simulink model "multi_model_attitude_controller1_1"  (R2016b)
settings: Solver=ode15s  StartTime=0.0  StopTime=inf  FixedStep=0.001  MaxStep=0.004  RelTol=1e-3
InitFcn:
  | kR_old=0;
  | kOm_old=0;
undefined symbols (not defined in the file or in its folder): deg, rad, s
libraries: simulink x32, aerolibconvert2 x6, aerolibobsolete x2, aerolibtransform2 x2, aerolibatmos2 x2, aerolibnav x2, aerolibanimutils x2
(part 2 of 3)

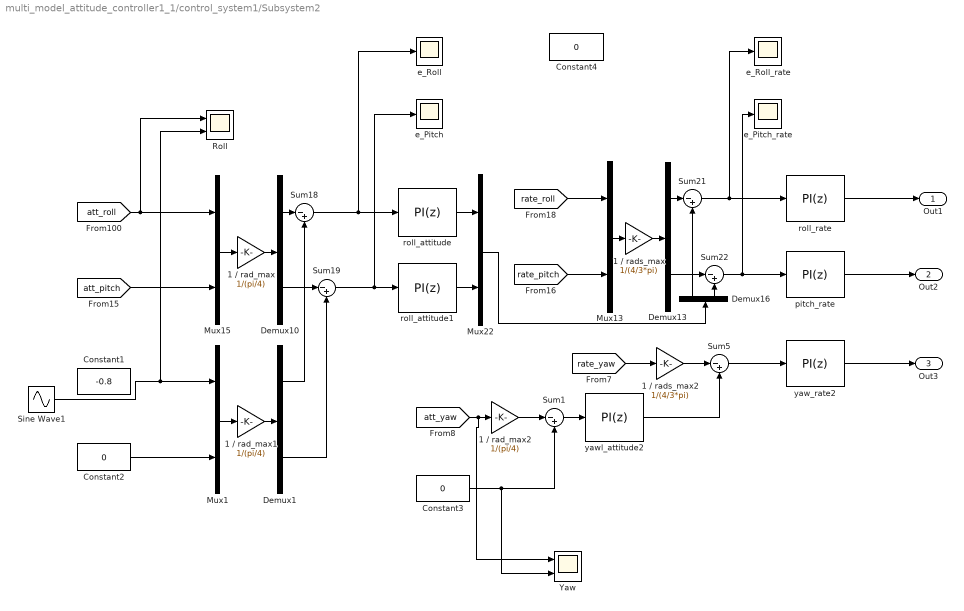
== system multi_model_attitude_controller1_1/control_system1/Subsystem2 ==
  1 / rad_max : Gain  Gain=1/(pi/4)
  1 / rad_max1 : Gain  Gain=1/(pi/4)
  1 / rad_max2 : Gain  Gain=1/(pi/4)
  1 / rads_max : Gain  Gain=1/(4/3*pi)
  1 / rads_max2 : Gain  Gain=1/(4/3*pi)
  Constant1 : Constant  Value=-0.8  SampleTime=0.004
  Constant2 : Constant  Value=0  SampleTime=0.004
  Constant3 : Constant  Value=0  SampleTime=0.004
  Constant4 : Constant  Value=0  SampleTime=0.004
  Demux{1,10,13,16} (4 alike) : Demux  Outputs=2
  Mux{1,13,15,22} (4 alike) : Mux  Inputs=2
  Roll : Scope  NumInputPorts=2
  Sine Wave1 : Sin  Amplitude=pi/9  Frequency=pi  Phase=pi/2  SampleTime=0.004
  Sum{1,5,18..19,21..22} (6 alike) : Sum  Inputs=|-+
  Yaw : Scope  NumInputPorts=2
  e_Pitch : Scope
  e_Pitch_rate : Scope
  e_Roll : Scope
  e_Roll_rate : Scope
  pitch_rate : simulink/Continuous/PID Controller  Controller=PI  TimeDomain=Discrete-time  SampleTime=-1  IntegratorMethod=Forward Euler  FilterMethod=Forward Euler  Form=Parallel  UseFilter=on  ControllerParametersSource=internal  P=0.266243984189179  I=1.55321106287276  D=0.0024  N=100  InitialConditionSource=internal  InitialConditionForIntegrator=0  InitialConditionForFilter=0  ExternalReset=none  LimitOutput=on  UpperSaturationLimit=1  LowerSaturationLimit=-1  LinearizeAsGain=on  AntiWindupMode=none  Kb=1  TrackingMode=off  Kt=1  PParamMin=[]  PParamMax=[]  IParamMin=[]  IParamMax=[]  DParamMin=[]  DParamMax=[]  NParamMin=[]  NParamMax=[]  KbParamMin=[]  KbParamMax=[]  KtParamMin=[]  KtParamMax=[]  POutMin=[]  POutMax=[]  IOutMin=[]  IOutMax=[]  DOutMin=[]  DOutMax=[]  NOutMin=[]  NOutMax=[]  KbOutMin=[]  KbOutMax=[]  KtOutMin=[]  KtOutMax=[]  IntegratorOutMin=[]  IntegratorOutMax=[]  FilterOutMin=[]  FilterOutMax=[]  SumOutMin=[]  SumOutMax=[]  SumI1OutMin=[]  SumI1OutMax=[]  SumI2OutMin=[]  SumI2OutMax=[]  SumI3OutMin=[]  SumI3OutMax=[]  SumDOutMin=[]  SumDOutMax=[]  SaturationOutMin=[]  SaturationOutMax=[]  IntegratorContinuousStateAttributes=''  IntegratorStateMustResolveToSignalObject=off  IntegratorRTWStateStorageClass=Auto  FilterContinuousStateAttributes=''  FilterStateMustResolveToSignalObject=off  FilterRTWStateStorageClass=Auto  DifferentiatorICPrevScaledInput=0  DifferentiatorOutMin=[]  DifferentiatorOutMax=[]
  roll_attitude : simulink/Continuous/PID Controller  Controller=PI  TimeDomain=Discrete-time  SampleTime=-1  IntegratorMethod=Forward Euler  FilterMethod=Forward Euler  Form=Parallel  UseFilter=on  ControllerParametersSource=internal  P=1.14248027715292  I=2.67479021353904  D=0.01  N=100  InitialConditionSource=internal  InitialConditionForIntegrator=0  InitialConditionForFilter=0  ExternalReset=none  LimitOutput=on  UpperSaturationLimit=1  LowerSaturationLimit=-1  LinearizeAsGain=on  AntiWindupMode=none  Kb=1  TrackingMode=off  Kt=1  PParamMin=[]  PParamMax=[]  IParamMin=[]  IParamMax=[]  DParamMin=[]  DParamMax=[]  NParamMin=[]  NParamMax=[]  KbParamMin=[]  KbParamMax=[]  KtParamMin=[]  KtParamMax=[]  POutMin=[]  POutMax=[]  IOutMin=[]  IOutMax=[]  DOutMin=[]  DOutMax=[]  NOutMin=[]  NOutMax=[]  KbOutMin=[]  KbOutMax=[]  KtOutMin=[]  KtOutMax=[]  IntegratorOutMin=[]  IntegratorOutMax=[]  FilterOutMin=[]  FilterOutMax=[]  SumOutMin=[]  SumOutMax=[]  SumI1OutMin=[]  SumI1OutMax=[]  SumI2OutMin=[]  SumI2OutMax=[]  SumI3OutMin=[]  SumI3OutMax=[]  SumDOutMin=[]  SumDOutMax=[]  SaturationOutMin=[]  SaturationOutMax=[]  IntegratorContinuousStateAttributes=''  IntegratorStateMustResolveToSignalObject=off  IntegratorRTWStateStorageClass=Auto  FilterContinuousStateAttributes=''  FilterStateMustResolveToSignalObject=off  FilterRTWStateStorageClass=Auto  DifferentiatorICPrevScaledInput=0  DifferentiatorOutMin=[]  DifferentiatorOutMax=[]
  roll_attitude1 : simulink/Continuous/PID Controller  Controller=PI  TimeDomain=Discrete-time  SampleTime=-1  IntegratorMethod=Forward Euler  FilterMethod=Forward Euler  Form=Parallel  UseFilter=on  ControllerParametersSource=internal  P=1.14248027709528  I=2.67479021340165  D=0.01  N=100  InitialConditionSource=internal  InitialConditionForIntegrator=0  InitialConditionForFilter=0  ExternalReset=none  LimitOutput=on  UpperSaturationLimit=1  LowerSaturationLimit=-1  LinearizeAsGain=on  AntiWindupMode=none  Kb=1  TrackingMode=off  Kt=1  PParamMin=[]  PParamMax=[]  IParamMin=[]  IParamMax=[]  DParamMin=[]  DParamMax=[]  NParamMin=[]  NParamMax=[]  KbParamMin=[]  KbParamMax=[]  KtParamMin=[]  KtParamMax=[]  POutMin=[]  POutMax=[]  IOutMin=[]  IOutMax=[]  DOutMin=[]  DOutMax=[]  NOutMin=[]  NOutMax=[]  KbOutMin=[]  KbOutMax=[]  KtOutMin=[]  KtOutMax=[]  IntegratorOutMin=[]  IntegratorOutMax=[]  FilterOutMin=[]  FilterOutMax=[]  SumOutMin=[]  SumOutMax=[]  SumI1OutMin=[]  SumI1OutMax=[]  SumI2OutMin=[]  SumI2OutMax=[]  SumI3OutMin=[]  SumI3OutMax=[]  SumDOutMin=[]  SumDOutMax=[]  SaturationOutMin=[]  SaturationOutMax=[]  IntegratorContinuousStateAttributes=''  IntegratorStateMustResolveToSignalObject=off  IntegratorRTWStateStorageClass=Auto  FilterContinuousStateAttributes=''  FilterStateMustResolveToSignalObject=off  FilterRTWStateStorageClass=Auto  DifferentiatorICPrevScaledInput=0  DifferentiatorOutMin=[]  DifferentiatorOutMax=[]
  roll_rate : simulink/Continuous/PID Controller  Controller=PI  TimeDomain=Discrete-time  SampleTime=-1  IntegratorMethod=Forward Euler  FilterMethod=Forward Euler  Form=Parallel  UseFilter=on  ControllerParametersSource=internal  P=0.327684903617463  I=1.91164438507472  D=0.0024  N=100  InitialConditionSource=internal  InitialConditionForIntegrator=0  InitialConditionForFilter=0  ExternalReset=none  LimitOutput=on  UpperSaturationLimit=1  LowerSaturationLimit=-1  LinearizeAsGain=on  AntiWindupMode=none  Kb=1  TrackingMode=off  Kt=1  PParamMin=[]  PParamMax=[]  IParamMin=[]  IParamMax=[]  DParamMin=[]  DParamMax=[]  NParamMin=[]  NParamMax=[]  KbParamMin=[]  KbParamMax=[]  KtParamMin=[]  KtParamMax=[]  POutMin=[]  POutMax=[]  IOutMin=[]  IOutMax=[]  DOutMin=[]  DOutMax=[]  NOutMin=[]  NOutMax=[]  KbOutMin=[]  KbOutMax=[]  KtOutMin=[]  KtOutMax=[]  IntegratorOutMin=[]  IntegratorOutMax=[]  FilterOutMin=[]  FilterOutMax=[]  SumOutMin=[]  SumOutMax=[]  SumI1OutMin=[]  SumI1OutMax=[]  SumI2OutMin=[]  SumI2OutMax=[]  SumI3OutMin=[]  SumI3OutMax=[]  SumDOutMin=[]  SumDOutMax=[]  SaturationOutMin=[]  SaturationOutMax=[]  IntegratorContinuousStateAttributes=''  IntegratorStateMustResolveToSignalObject=off  IntegratorRTWStateStorageClass=Auto  FilterContinuousStateAttributes=''  FilterStateMustResolveToSignalObject=off  FilterRTWStateStorageClass=Auto  DifferentiatorICPrevScaledInput=0  DifferentiatorOutMin=[]  DifferentiatorOutMax=[]
  yaw_rate2 : simulink/Continuous/PID Controller  Controller=PI  TimeDomain=Discrete-time  SampleTime=-1  IntegratorMethod=Forward Euler  FilterMethod=Forward Euler  Form=Parallel  UseFilter=on  ControllerParametersSource=internal  P=0.3  I=0.03  D=0.0024  N=100  InitialConditionSource=internal  InitialConditionForIntegrator=0  InitialConditionForFilter=0  ExternalReset=none  LimitOutput=on  UpperSaturationLimit=1  LowerSaturationLimit=-1  LinearizeAsGain=on  AntiWindupMode=none  Kb=1  TrackingMode=off  Kt=1  PParamMin=[]  PParamMax=[]  IParamMin=[]  IParamMax=[]  DParamMin=[]  DParamMax=[]  NParamMin=[]  NParamMax=[]  KbParamMin=[]  KbParamMax=[]  KtParamMin=[]  KtParamMax=[]  POutMin=[]  POutMax=[]  IOutMin=[]  IOutMax=[]  DOutMin=[]  DOutMax=[]  NOutMin=[]  NOutMax=[]  KbOutMin=[]  KbOutMax=[]  KtOutMin=[]  KtOutMax=[]  IntegratorOutMin=[]  IntegratorOutMax=[]  FilterOutMin=[]  FilterOutMax=[]  SumOutMin=[]  SumOutMax=[]  SumI1OutMin=[]  SumI1OutMax=[]  SumI2OutMin=[]  SumI2OutMax=[]  SumI3OutMin=[]  SumI3OutMax=[]  SumDOutMin=[]  SumDOutMax=[]  SaturationOutMin=[]  SaturationOutMax=[]  IntegratorContinuousStateAttributes=''  IntegratorStateMustResolveToSignalObject=off  IntegratorRTWStateStorageClass=Auto  FilterContinuousStateAttributes=''  FilterStateMustResolveToSignalObject=off  FilterRTWStateStorageClass=Auto  DifferentiatorICPrevScaledInput=0  DifferentiatorOutMin=[]  DifferentiatorOutMax=[]
  yawl_attitude2 : simulink/Continuous/PID Controller  Controller=PI  TimeDomain=Discrete-time  SampleTime=-1  IntegratorMethod=Forward Euler  FilterMethod=Forward Euler  Form=Parallel  UseFilter=on  ControllerParametersSource=internal  P=0.5  I=0.05  D=0.01  N=100  InitialConditionSource=internal  InitialConditionForIntegrator=0  InitialConditionForFilter=0  ExternalReset=none  LimitOutput=on  UpperSaturationLimit=1  LowerSaturationLimit=-1  LinearizeAsGain=on  AntiWindupMode=none  Kb=1  TrackingMode=off  Kt=1  PParamMin=[]  PParamMax=[]  IParamMin=[]  IParamMax=[]  DParamMin=[]  DParamMax=[]  NParamMin=[]  NParamMax=[]  KbParamMin=[]  KbParamMax=[]  KtParamMin=[]  KtParamMax=[]  POutMin=[]  POutMax=[]  IOutMin=[]  IOutMax=[]  DOutMin=[]  DOutMax=[]  NOutMin=[]  NOutMax=[]  KbOutMin=[]  KbOutMax=[]  KtOutMin=[]  KtOutMax=[]  IntegratorOutMin=[]  IntegratorOutMax=[]  FilterOutMin=[]  FilterOutMax=[]  SumOutMin=[]  SumOutMax=[]  SumI1OutMin=[]  SumI1OutMax=[]  SumI2OutMin=[]  SumI2OutMax=[]  SumI3OutMin=[]  SumI3OutMax=[]  SumDOutMin=[]  SumDOutMax=[]  SaturationOutMin=[]  SaturationOutMax=[]  IntegratorContinuousStateAttributes=''  IntegratorStateMustResolveToSignalObject=off  IntegratorRTWStateStorageClass=Auto  FilterContinuousStateAttributes=''  FilterStateMustResolveToSignalObject=off  FilterRTWStateStorageClass=Auto  DifferentiatorICPrevScaledInput=0  DifferentiatorOutMin=[]  DifferentiatorOutMax=[]
  Out1 : Outport
  Out2 : Outport  Port=2
  Out3 : Outport  Port=3
  wires:
  Sine Wave1/1 -> Roll/2, Mux1/1
  Mux1/1 -> 1 / rad_max1/1
  Constant2/1 -> Mux1/2
  Demux1/1 -> Sum18/2
  Mux22/1 -> Demux16/1
  yaw_rate2/1 -> Out3/1
  Sum5/1 -> yaw_rate2/1
  yawl_attitude2/1 -> Sum5/2
  1 / rad_max2/1 -> Sum1/1
  [att_yaw] -> Yaw/1, 1 / rad_max2/1
  1 / rads_max2/1 -> Sum5/1
  [rate_yaw] -> 1 / rads_max2/1
  1 / rad_max/1 -> Demux10/1
  Demux10/1 -> Sum18/1
  Demux16/2 -> Sum22/2
  roll_attitude1/1 -> Mux22/2
  Demux13/2 -> Sum22/1
  Sum21/1 -> e_Roll_rate/1, roll_rate/1
  Sum22/1 -> e_Pitch_rate/1, pitch_rate/1
  roll_attitude/1 -> Mux22/1
  [rate_pitch] -> Mux13/2
  Demux10/2 -> Sum19/1
  [att_pitch] -> Mux15/2
  [rate_roll] -> Mux13/1
  1 / rads_max/1 -> Demux13/1
  Sum18/1 -> e_Roll/1, roll_attitude/1
  Mux13/1 -> 1 / rads_max/1
  Demux13/1 -> Sum21/1
  Sum19/1 -> e_Pitch/1, roll_attitude1/1
  Mux15/1 -> 1 / rad_max/1
  [att_roll] -> Roll/1, Mux15/1
  roll_rate/1 -> Out1/1
  pitch_rate/1 -> Out2/1
  1 / rad_max1/1 -> Demux1/1
  Demux1/2 -> Sum19/2
  Sum1/1 -> yawl_attitude2/1
  Constant3/1 -> Yaw/2, Sum1/2
  Demux16/1 -> Sum21/2

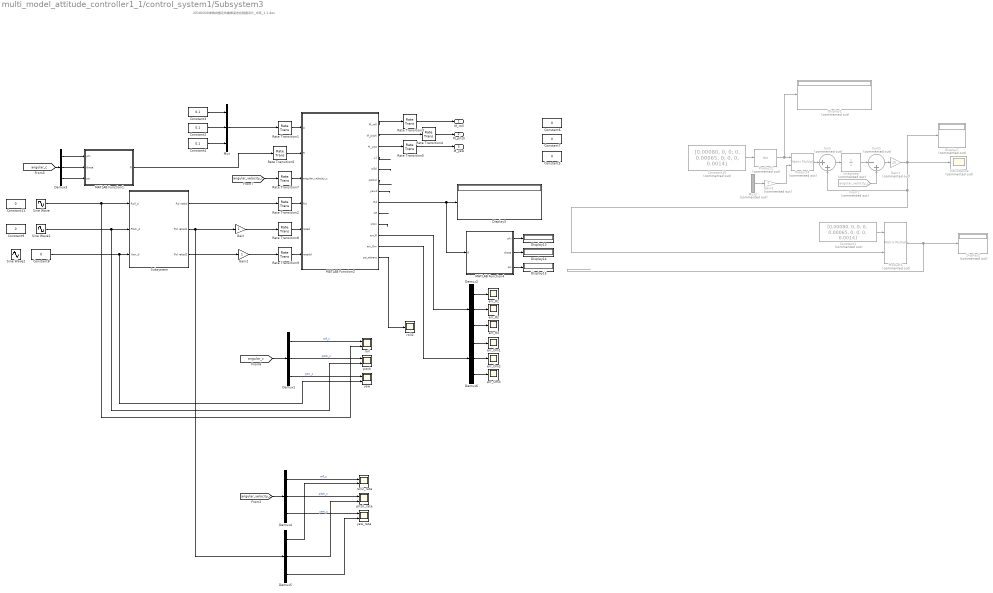
== system multi_model_attitude_controller1_1/control_system1/Subsystem3 ==
  note: 20180328 参数自整定的鲁棒姿态控制器设计_中英_1.1.doc
  Constant1 : Constant  Commented=on  Value=[0.00080, 0, 0; 0, 0.00065, 0; 0, 0, 0.0014]  SampleTime=0.004
  Constant10 : Constant  Commented=on  Value=[0.00080, 0, 0; 0, 0.00065, 0; 0, 0, 0.0014]  SampleTime=0.004
  Constant{5..9,11} (6 alike) : Constant  Value=0  SampleTime=0.004
  Constant2 : Constant  Value=0.1  SampleTime=0.004
  Constant3 : Constant  Value=0.1  SampleTime=0.004
  Constant4 : Constant  Value=0.1  SampleTime=0.004
  Demux{1..6} (6 alike) : Demux  Outputs=3
  Display1 : Display  Commented=on
  Display{3,13..15} (4 alike) : Display
  Display2 : Display  Commented=on
  Display7 : Display  Commented=on
  From1 : From  Commented=on  GotoTag=angular_velocity_c  TagVisibility=global
  Gain : Gain
  Gain1 : Gain  Commented=on  Gain=20
  Gain2 : Gain
  Gain3 : Gain  Commented=on
  Integrator : Integrator  Commented=on
  MATLAB Function1 : MATLAB Function  TreatAsAtomicUnit=on
  MATLAB Function2 : MATLAB Function  TreatAsAtomicUnit=on
  MATLAB Function4 : MATLAB Function  TreatAsAtomicUnit=on
  Mux : Mux  Inputs=3
  Mux2 : Mux  Commented=on  Inputs=3
  Product1 : Product  Commented=on  Multiplication=Matrix(*)
  Product2 : Product  Commented=on  Inputs=/  Multiplication=Matrix(*)
  Product4 : Product  Commented=on  Multiplication=Matrix(*)
  Rate Transition{1..9} (9 alike) : RateTransition  OutPortSampleTime=0.004
  Sine Wave : Sin  Amplitude=pi/9  Frequency=pi  SampleTime=0.004
  Sine Wave1 : Sin  Amplitude=pi/9  Frequency=pi  Phase=pi/2  SampleTime=0.004
  Sine Wave2 : Sin  Amplitude=pi/9  Frequency=pi  SampleTime=0.004
  Subsystem : Subsystem
  Sum : Sum  Commented=on  Inputs=|++
  Sum1 : Sum  Commented=on  Inputs=|-+
  disturbance : Scope  Commented=on
  err_Om1 : Scope
  err_Om2 : Scope
  err_Om3 : Scope
  err_R1 : Scope
  err_R2 : Scope
  err_R3 : Scope
  pitch : Scope  NumInputPorts=2
  pitch_rate : Scope  NumInputPorts=2
  roll : Scope  NumInputPorts=2
  roll2 : Scope
  roll2_rate : Scope  NumInputPorts=2
  yaw : Scope  NumInputPorts=2
  yaw_rate : Scope  NumInputPorts=2
  M_roll : Outport
  M_pitch : Outport  Port=2
  M_yaw : Outport  Port=3
  wires:
  Gain3/1 -> Product4/2
  Product1/1 -> Display2/1
  Rate Transition5/1 -> M_yaw/1
  Rate Transition4/1 -> M_pitch/1
  Rate Transition3/1 -> M_roll/1
  Constant1/1 -> Product1/1
  Rate Transition2/1 -> MATLAB Function2/4("Rd ")
  Constant2/1 -> Mux/2
  From1/1 -> Sum1/2
  Gain1/1 -> Display7/1, disturbance/1, Sum/2, Product1/2
  Mux/1 -> Rate Transition1/1
  Constant10/1 -> Product2/1
  Product2/1 -> Product4/1, Display1/1
  MATLAB Function2/3(M_yaw) -> Rate Transition5/1
  Sine Wave/1 -> roll/2, Subsystem/1(Roll_d)
  Sum1/1 -> Gain1/1
  MATLAB Function2/1(M_roll) -> Rate Transition3/1
  Sum/1 -> Integrator/1
  Product4/1 -> Sum/1
  Constant3/1 -> Mux/1
  MATLAB Function2/2(M_pitch) -> Rate Transition4/1
  Subsystem/1(Rd rated) -> Rate Transition2/1
  Constant4/1 -> Mux/3
  Mux2/1 -> Gain3/1
  Integrator/1 -> Sum1/1
  Rate Transition6/1 -> MATLAB Function2/2(R)
  Demux1/3 -> yaw/1  "yaw_c"
  Rate Transition7/1 -> MATLAB Function2/3(angular_velocity_c)
  Demux1/1 -> roll/1  "roll_c"
  Rate Transition1/1 -> MATLAB Function2/1(A)
  [angular_velocity_c] -> Rate Transition7/1
  MATLAB Function1/1(R) -> Rate Transition6/1
  Demux1/2 -> pitch/1  "pitch_c"
  MATLAB Function2/5(rolld) -> ?
  MATLAB Function2/7(yawd) -> ?
  MATLAB Function2/6(pitchd) -> ?
  MATLAB Function2/4(u1) -> ?
  Demux2/1 -> err_R1/1
  MATLAB Function2/9(kR) -> ?
  MATLAB Function2/10(kOm) -> ?
  Demux2/2 -> err_R2/1
  Demux2/3 -> err_R3/1
  Constant8/1 -> yaw/2, Subsystem/3(Yaw_d)
  Sine Wave1/1 -> pitch/2, Subsystem/2(PItch_d)
  MATLAB Function4/1(phi) -> Display13/1
  MATLAB Function4/2(theta) -> Display14/1
  MATLAB Function4/3(psi) -> Display15/1
  MATLAB Function2/8(Rd) -> MATLAB Function4/1(R), Display3/1
  [angular_c] -> Demux1/1
  Demux3/2 -> MATLAB Function1/2(theta)
  Demux3/1 -> MATLAB Function1/1(phi)
  Demux3/3 -> MATLAB Function1/3(psi)
  Rate Transition8/1 -> MATLAB Function2/5(rated)
  Rate Transition9/1 -> MATLAB Function2/6(ratedd)
  Subsystem/2(Rd rated1) -> Demux5/1, Gain/1
  Subsystem/3(Rd rated2) -> Gain2/1
  Demux4/3 -> yaw_rate/1  "yaw_c"
  Demux4/1 -> roll2_rate/1  "roll_c"
  Demux4/2 -> pitch_rate/1  "pitch_c"
  [angular_velocity_c] -> Demux4/1
  Demux5/1 -> roll2_rate/2
  Demux5/2 -> pitch_rate/2
  Demux5/3 -> yaw_rate/2
  [angular_c] -> Demux3/1
  MATLAB Function2/13(psi_attract) -> roll2/1
  MATLAB Function2/11(err_R) -> Demux2/1
  Demux6/1 -> err_Om1/1
  Demux6/2 -> err_Om2/1
  Demux6/3 -> err_Om3/1
  MATLAB Function2/12(err_Om) -> Demux6/1
  Gain/1 -> Rate Transition8/1
  Gain2/1 -> Rate Transition9/1

== system multi_model_attitude_controller1_1/dynamic_model1/normalize ==
  pwm1 : Inport
  pwm2 : Inport  Port=2
  pwm3 : Inport  Port=3
  pwm4 : Inport  Port=4
  pwm5 : Inport  Port=5
  pwm6 : Inport  Port=6
  pwm7 : Inport  Port=7
  pwm8 : Inport  Port=8
  Mux5 : Mux  Inputs=8
  Saturation{,3..9} (8 alike) : Saturate  UpperLimit=1  LowerLimit=0
  voltage{1..8} (8 alike) : Fcn  Expr=(u-1000)/1000
  normalized_signals : Outport
  wires:
  Saturation5/1 -> Mux5/4
  Saturation7/1 -> Mux5/6
  voltage6/1 -> Saturation7/1
  voltage5/1 -> Saturation5/1
  voltage2/1 -> Saturation/1
  voltage7/1 -> Saturation8/1
  Saturation8/1 -> Mux5/7
  voltage8/1 -> Saturation9/1
  Saturation9/1 -> Mux5/8
  pwm3/1 -> voltage4/1
  Mux5/1 -> normalized_signals/1
  pwm1/1 -> voltage2/1
  voltage4/1 -> Saturation4/1
  Saturation4/1 -> Mux5/3
  pwm7/1 -> voltage7/1
  pwm6/1 -> voltage6/1
  pwm8/1 -> voltage8/1
  pwm4/1 -> voltage5/1
  pwm5/1 -> voltage1/1
  pwm2/1 -> voltage3/1
  voltage1/1 -> Saturation6/1
  Saturation6/1 -> Mux5/5
  Saturation/1 -> Mux5/1
  Saturation3/1 -> Mux5/2
  voltage3/1 -> Saturation3/1

== system multi_model_attitude_controller1_1/dynamic_model1/transfer_function ==
  load : Inport  PortDimensions=[8]
  voltage : Inport  Port=2  PortDimensions=[8]
  Demux13 : Demux  Outputs=8
  Mux4 : Mux  Inputs=8
  Product : Product
  Transfer Fcn{1..8} (8 alike) : TransferFcn  Numerator=[325]  Denominator=[2.5e-08 0.01 1]  ContinuousStateAttributes='angular_velocity'
  thrust : Outport
  wires:
  Demux13/6 -> Transfer Fcn6/1
  Transfer Fcn4/1 -> Mux4/4
  Transfer Fcn2/1 -> Mux4/3
  Demux13/8 -> Transfer Fcn8/1
  Transfer Fcn8/1 -> Mux4/8
  Transfer Fcn1/1 -> Mux4/2
  Demux13/7 -> Transfer Fcn7/1
  Transfer Fcn7/1 -> Mux4/7
  Transfer Fcn5/1 -> Mux4/5
  Demux13/5 -> Transfer Fcn5/1
  Transfer Fcn3/1 -> Mux4/1
  Transfer Fcn6/1 -> Mux4/6
  Demux13/1 -> Transfer Fcn3/1
  Demux13/2 -> Transfer Fcn1/1
  Demux13/3 -> Transfer Fcn2/1
  Demux13/4 -> Transfer Fcn4/1
  voltage/1 -> Product/2
  Product/1 -> Demux13/1
  Mux4/1 -> thrust/1
  load/1 -> Product/1

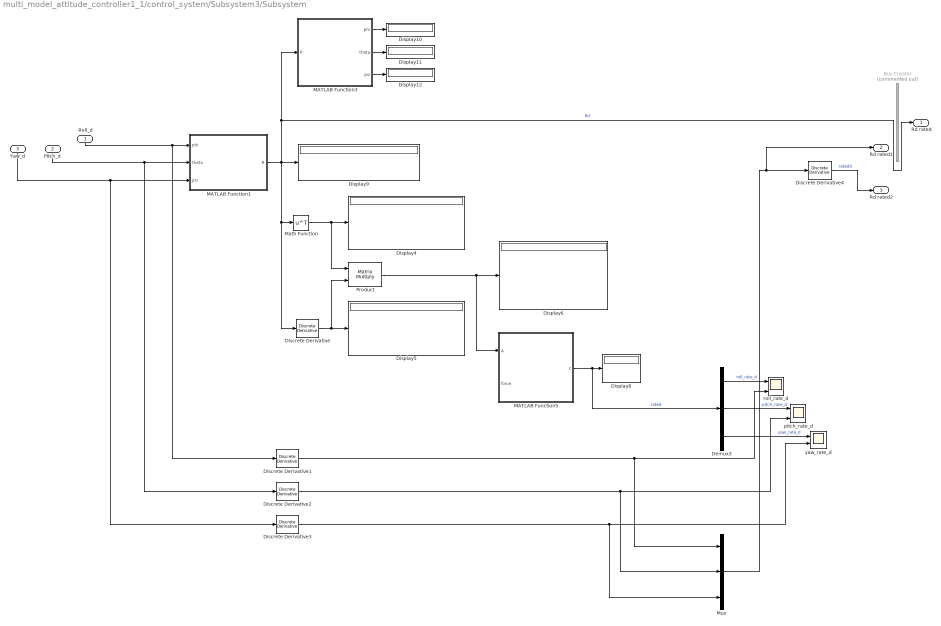
== system multi_model_attitude_controller1_1/control_system/Subsystem3/Subsystem ==
  Roll_d : Inport
  PItch_d : Inport  Port=2
  Yaw_d : Inport  Port=3
  Bus Creator : BusCreator  Commented=on  Inputs=3
  Demux3 : Demux  Outputs=3
  Discrete Derivative{,1..4} (5 alike) : simulink/Discrete/Discrete Derivative  gainval=1.0  ICPrevScaledInput=0.0  OutMin=[]  OutMax=[]  OutDataType=fixdt(1, 16)  OutScaling=2^-10  DoSatur=off
  Display{4..6,8..12} (8 alike) : Display
  MATLAB Function1 : MATLAB Function  TreatAsAtomicUnit=on
  MATLAB Function3 : MATLAB Function  TreatAsAtomicUnit=on
  MATLAB Function5 : MATLAB Function  TreatAsAtomicUnit=on
  Math Function : Math  Operator=transpose  SaturateOnIntegerOverflow=on
  Mux : Mux  Inputs=3
  Product : Product  Multiplication=Matrix(*)
  pitch_rate_d : Scope  NumInputPorts=2
  roll_rate_d : Scope  NumInputPorts=2
  yaw_rate_d : Scope  NumInputPorts=2
  Rd rated : Outport
  Rd rated1 : Outport  Port=2
  Rd rated2 : Outport  Port=3
  wires:
  Discrete Derivative3/1 -> yaw_rate_d/2, Mux/3
  MATLAB Function3/2(theta) -> Display11/1
  Discrete Derivative1/1 -> roll_rate_d/2, Mux/1
  Discrete Derivative2/1 -> pitch_rate_d/2, Mux/2
  Product/1 -> MATLAB Function5/1(A), Display6/1
  Discrete Derivative/1 -> Product/2, Display5/1
  MATLAB Function1/1(R) -> Rd rated/1, MATLAB Function3/1(R), Display9/1, Math Function/1, Discrete Derivative/1  "Rd"
  MATLAB Function3/1(phi) -> Display10/1
  MATLAB Function3/3(psi) -> Display12/1
  Math Function/1 -> Product/1, Display4/1
  MATLAB Function5/1(t) -> Demux3/1, Display8/1  "rated"
  Demux3/3 -> yaw_rate_d/1  "yaw_rate_d"
  Demux3/1 -> roll_rate_d/1  "roll_rate_d"
  Demux3/2 -> pitch_rate_d/1  "pitch_rate_d"
  Roll_d/1 -> Discrete Derivative1/1, MATLAB Function1/1(phi)
  ? -> MATLAB Function5/2(force)
  Yaw_d/1 -> Discrete Derivative3/1, MATLAB Function1/3(psi)
  PItch_d/1 -> Discrete Derivative2/1, MATLAB Function1/2(theta)
  Discrete Derivative4/1 -> Rd rated2/1  "ratedd"
  Mux/1 -> Rd rated1/1, Discrete Derivative4/1

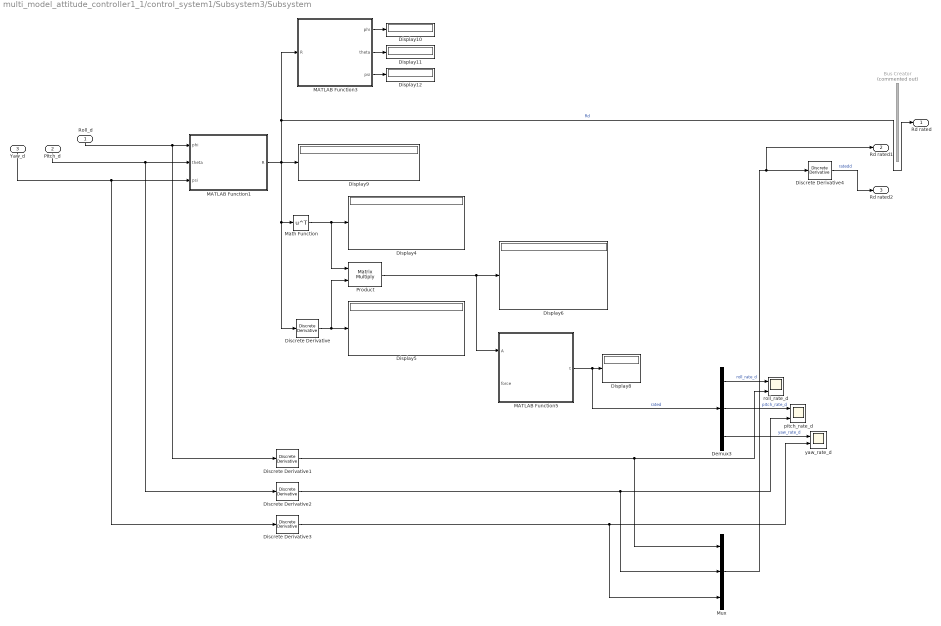
== system multi_model_attitude_controller1_1/control_system1/Subsystem3/Subsystem ==
  Roll_d : Inport
  PItch_d : Inport  Port=2
  Yaw_d : Inport  Port=3
  Bus Creator : BusCreator  Commented=on  Inputs=3
  Demux3 : Demux  Outputs=3
  Discrete Derivative{,1..4} (5 alike) : simulink/Discrete/Discrete Derivative  gainval=1.0  ICPrevScaledInput=0.0  OutMin=[]  OutMax=[]  OutDataType=fixdt(1, 16)  OutScaling=2^-10  DoSatur=off
  Display{4..6,8..12} (8 alike) : Display
  MATLAB Function1 : MATLAB Function  TreatAsAtomicUnit=on
  MATLAB Function3 : MATLAB Function  TreatAsAtomicUnit=on
  MATLAB Function5 : MATLAB Function  TreatAsAtomicUnit=on
  Math Function : Math  Operator=transpose  SaturateOnIntegerOverflow=on
  Mux : Mux  Inputs=3
  Product : Product  Multiplication=Matrix(*)
  pitch_rate_d : Scope  NumInputPorts=2
  roll_rate_d : Scope  NumInputPorts=2
  yaw_rate_d : Scope  NumInputPorts=2
  Rd rated : Outport
  Rd rated1 : Outport  Port=2
  Rd rated2 : Outport  Port=3
  wires:
  Discrete Derivative3/1 -> yaw_rate_d/2, Mux/3
  MATLAB Function3/2(theta) -> Display11/1
  Discrete Derivative1/1 -> roll_rate_d/2, Mux/1
  Discrete Derivative2/1 -> pitch_rate_d/2, Mux/2
  Product/1 -> MATLAB Function5/1(A), Display6/1
  Discrete Derivative/1 -> Product/2, Display5/1
  MATLAB Function1/1(R) -> Rd rated/1, MATLAB Function3/1(R), Display9/1, Math Function/1, Discrete Derivative/1  "Rd"
  MATLAB Function3/1(phi) -> Display10/1
  MATLAB Function3/3(psi) -> Display12/1
  Math Function/1 -> Product/1, Display4/1
  MATLAB Function5/1(t) -> Demux3/1, Display8/1  "rated"
  Demux3/3 -> yaw_rate_d/1  "yaw_rate_d"
  Demux3/1 -> roll_rate_d/1  "roll_rate_d"
  Demux3/2 -> pitch_rate_d/1  "pitch_rate_d"
  Roll_d/1 -> Discrete Derivative1/1, MATLAB Function1/1(phi)
  ? -> MATLAB Function5/2(force)
  Yaw_d/1 -> Discrete Derivative3/1, MATLAB Function1/3(psi)
  PItch_d/1 -> Discrete Derivative2/1, MATLAB Function1/2(theta)
  Discrete Derivative4/1 -> Rd rated2/1  "ratedd"
  Mux/1 -> Rd rated1/1, Discrete Derivative4/1

== matlab function multi_model_attitude_controller1_1/dynamic_model/MATLAB Function ==
  data: roll input; pitch input; altitude input; sonar_alt output
function sonar_alt = ultrasonic(roll, pitch, altitude)
if altitude > 0
    sonar_alt = sqrt(altitude^2 + (sqrt((altitude*tan(roll))^2 + (altitude*tan(pitch))^2))^2);
else
    sonar_alt = 0;
end

== matlab function multi_model_attitude_controller1_1/control_system1/Subsystem/MATLAB Function3 ==
  data: angular input; R output
function R = RPY_2_ZXY(angular)
%written by Daniel Mellinger
phi=angular(1);theta=angular(2);psi=angular(3);
% BRW = [ cos(psi)*cos(theta) - sin(phi)*sin(psi)*sin(theta), 
%     cos(theta)*sin(psi) + cos(psi)*sin(phi)*sin(theta), -cos(phi)*sin(theta)]
% 
% [                                 -cos(phi)*sin(psi),
%     cos(phi)*cos(psi),             sin(phi)]
% 
% [ cos(psi)*sin(theta) + cos(theta)*sin(phi)*sin(psi), 
%     sin(psi)*sin(theta) - cos(psi)*cos(theta)*sin(phi),
%     cos(phi)*cos(theta)]

R = [ cos(psi)*cos(theta) - sin(phi)*sin(psi)*sin(theta),... 
    cos(theta)*sin(psi) + cos(psi)*sin(phi)*sin(theta), -cos(phi)*sin(theta);...
    -cos(phi)*sin(psi),...
    cos(phi)*cos(psi),             sin(phi);...
    cos(psi)*sin(theta) + cos(theta)*sin(phi)*sin(psi),...
    sin(psi)*sin(theta) - cos(psi)*cos(theta)*sin(phi),...
    cos(phi)*cos(theta)];
    
    R = R';

== matlab function multi_model_attitude_controller1_1/control_system/Subsystem3/MATLAB Function2 ==
  data: A input; M_roll output; R input; angular_velocity_c input; M_pitch output; M_yaw output; u1 output; rolld output; pitchd output; yawd output; Rd output; kR output; kOm output; Rd input; err_R output; err_Om output; rated input; ratedd input; psi_attract output
function [M_roll, M_pitch,M_yaw,u1,rolld,pitchd,yawd,Rd,kR,kOm,err_R,err_Om,psi_attract] = attitude(A,R,angular_velocity_c,Rd,rated,ratedd)

 J = diag([0.00080, 0.00065, 0.0014]);
 J_ni=inv(J);
 e1 = [1;0;0];e2 = [0;1;0];e3 = [0;0;1];

Omega=angular_velocity_c;

Omegad = rated;
dOmegad = ratedd;

 b3c = A/norm(A);
 b3 = R(:,3);
 f = vec_dot(A,b3);
 u1=f;
    
%%%%%  姿态控制
 b1d = e1;
 b1c = -vec_cross(b3c,vec_cross(b3c,b1d));
 b1c = b1c/norm(vec_cross(b3c,b1d));
 Rc = [b1c vec_cross(b3c,b1c) b3c];
 

[rolld,pitchd,yawd]=RotToRPY_ZXY(Rd);
 if(norm(Rd'*Rd-eye(3)) > 1e-2)
        disp('Error in R') ;
 end

%  kR = 0.4 ; kOm = 0.4 ;
%   kR = 3	 ; kOm =2 ;
%   kR = 0.09	 ; kOm =1 ;
kR = 0.001	 ; kOm =0;
% epsilon = 0.1 ; %.5 ; %0.01 ;

psi_attract = 1/2*trace(eye(3,3)-Rd'*R);
err_R = 1/2 * vee_map(Rd'*R - R'*Rd) ;
err_Om = Omega - R'*Rd*Omegad ;
 

% % kR=0.1.*kR+err_R'*err_Om;
% % if kR>1
% %     kR=1;
% % end
% % if kR<-1
% %     kR=-1;
% % end
% % 
% % kOm=0.1.*kOm+0.01.*err_R'*err_Om;
% % if kOm>0.5
% %     kOm=0.5;
% % end
% % if kOm<-0.5
% %     kOm=0-0.5;
% % end

c2=0.02;
eA=err_Om+c2.*J_ni*err_R;
deltaR=0.3;
sigamaR=0.01;
k=0.1;

miu=-(deltaR.^2+k.*sigamaR).*eA./(deltaR*norm(eA)+sigamaR);
% miu=[0;0;0];


% % M = -kR.*err_R - kOm.*err_Om+ vec_cross(Omega, J*Omega)- J*(hat_map(Omega)*R'*Rd*Omegad - R'*Rd*dOmegad)+miu ;
M = -kR.*err_R - kOm.*err_Om+ vec_cross(Omega, J*Omega)- J*(hat_map(Omega)*R'*Rd*Omegad - R'*Rd*dOmegad);
M_roll=M(1);M_pitch=M(2);M_yaw=M(3);

== matlab function multi_model_attitude_controller1_1/control_system/Subsystem3/Subsystem/MATLAB Function5 ==
  data: A input; t output; force input
function t = vee_map(A, force)
    if(nargin == 1)
        force = false ;
    end
    if(~force)
        if(double(sum(abs(diag(A)))) > 1e-2)
            disp('Error in vee_map() - Nonzero diagonal') ;
%             keyboard ;
        end
    end
    %A = [0 -t(3) t(2) ; t(3) 0 -t(1) ; -t(2) t(1) 0] ;
    t = [A(3,2) ;
         A(1,3) ;
         A(2,1)] ;
end

== matlab function multi_model_attitude_controller1_1/control_system/Subsystem1/MATLAB Function2 ==
  data: A input; M_roll output; angular_c input; angular_velocity_c input; M_pitch output; M_yaw output; u1 output; rolld output; pitchd output; yawd output; angular_d input; disturbance input
function [M_roll, M_pitch,M_yaw,u1,rolld,pitchd,yawd] = attitude(A,angular_c,angular_velocity_c,angular_d,disturbance)

 J = diag([0.00080, 0.00065, 0.0014]);
 e1 = [1;0;0];e2 = [0;1;0];e3 = [0;0;1];
%%当前状态量
roll=angular_c(1);pitch=angular_c(2);yaw=angular_c(3);

R= RPYtoRot_ZXY(roll,pitch,yaw);
Omega=angular_velocity_c;

 b3c = A/norm(A);
 b3 = R(:,3);
 f = vec_dot(A,b3);
 u1=f;
    
%%%%%  姿态控制
 b1d = e1;
 b1c = -vec_cross(b3c,vec_cross(b3c,b1d));
 b1c = b1c/norm(vec_cross(b3c,b1d));
 Rc = [b1c vec_cross(b3c,b1c) b3c];
 
roll_d=pi/4;
pitch_d=-pi/4;
yaw_d=0;

roll_d=angular_d(1);
pitch_d=angular_d(2);
yaw_d=angular_d(3);

Rc= RPYtoRot_ZXY(roll_d,pitch_d,yaw_d);
Rd = Rc;
[rolld,pitchd,yawd]=RotToRPY_ZXY(Rd);
 if(norm(Rd'*Rd-eye(3)) > 1e-2)
        disp('Error in R') ;
 end

%  kR = 0.4 ; kOm = 0.4 ;
%   kR = 3	 ; kOm =2 ;
%   kR = 0.09	 ; kOm =1 ;
kR = 4	 ; kOm =1 ;
% epsilon = 0.1 ; %.5 ; %0.01 ;
Omegad = zeros(3,1);
dOmegad = zeros(3,1);
err_R = 1/2 * vee_map(Rd'*R - R'*Rd) ;
err_Om = Omega - R'*Rd*Omegad ;
 
% M = -kR.*err_R - kOm.*err_Om+ vec_cross(Omega, J*Omega)- J*(hat_map(Omega)*R'*Rd*Omegad - R'*Rd*dOmegad) ;
M = -kR.*err_R - kOm.*err_Om+ vec_cross(Omega, J*Omega)- J*(hat_map(Omega)*R'*Rd*Omegad - R'*Rd*dOmegad)-(disturbance) ;
M_roll=M(1);M_pitch=M(2);M_yaw=M(3);
% M_phi=0 ;M_theta=0;M_psi=0;
% M_pitch=0;
% % M_roll=0 ;
% M_yaw=0;
% u1=0.5;

== matlab function multi_model_attitude_controller1_1/control_system1/Subsystem/MATLAB Function4 ==
  data: angular input; R output
function R = RPY_2_ZXY(angular)
%written by Daniel Mellinger
phi=angular(1);theta=angular(2);psi=angular(3);
% BRW = [ cos(psi)*cos(theta) - sin(phi)*sin(psi)*sin(theta), 
%     cos(theta)*sin(psi) + cos(psi)*sin(phi)*sin(theta), -cos(phi)*sin(theta)]
% 
% [                                 -cos(phi)*sin(psi),
%     cos(phi)*cos(psi),             sin(phi)]
% 
% [ cos(psi)*sin(theta) + cos(theta)*sin(phi)*sin(psi), 
%     sin(psi)*sin(theta) - cos(psi)*cos(theta)*sin(phi),
%     cos(phi)*cos(theta)]

R = [ cos(psi)*cos(theta) - sin(phi)*sin(psi)*sin(theta),... 
    cos(theta)*sin(psi) + cos(psi)*sin(phi)*sin(theta), -cos(phi)*sin(theta);...
    -cos(phi)*sin(psi),...
    cos(phi)*cos(psi),             sin(phi);...
    cos(psi)*sin(theta) + cos(theta)*sin(phi)*sin(psi),...
    sin(psi)*sin(theta) - cos(psi)*cos(theta)*sin(phi),...
    cos(phi)*cos(theta)];
    
    R = R';

== matlab function multi_model_attitude_controller1_1/control_system/Subsystem/MATLAB Function3 ==
  data: angular input; R output
function R = RPY_2_ZXY(angular)
%written by Daniel Mellinger
phi=angular(1);theta=angular(2);psi=angular(3);
% BRW = [ cos(psi)*cos(theta) - sin(phi)*sin(psi)*sin(theta), 
%     cos(theta)*sin(psi) + cos(psi)*sin(phi)*sin(theta), -cos(phi)*sin(theta)]
% 
% [                                 -cos(phi)*sin(psi),
%     cos(phi)*cos(psi),             sin(phi)]
% 
% [ cos(psi)*sin(theta) + cos(theta)*sin(phi)*sin(psi), 
%     sin(psi)*sin(theta) - cos(psi)*cos(theta)*sin(phi),
%     cos(phi)*cos(theta)]

R = [ cos(psi)*cos(theta) - sin(phi)*sin(psi)*sin(theta),... 
    cos(theta)*sin(psi) + cos(psi)*sin(phi)*sin(theta), -cos(phi)*sin(theta);...
    -cos(phi)*sin(psi),...
    cos(phi)*cos(psi),             sin(phi);...
    cos(psi)*sin(theta) + cos(theta)*sin(phi)*sin(psi),...
    sin(psi)*sin(theta) - cos(psi)*cos(theta)*sin(phi),...
    cos(phi)*cos(theta)];
    
    R = R';

== matlab function multi_model_attitude_controller1_1/control_system/Subsystem/MATLAB Function4 ==
  data: angular input; R output
function R = RPY_2_ZXY(angular)
%written by Daniel Mellinger
phi=angular(1);theta=angular(2);psi=angular(3);
% BRW = [ cos(psi)*cos(theta) - sin(phi)*sin(psi)*sin(theta), 
%     cos(theta)*sin(psi) + cos(psi)*sin(phi)*sin(theta), -cos(phi)*sin(theta)]
% 
% [                                 -cos(phi)*sin(psi),
%     cos(phi)*cos(psi),             sin(phi)]
% 
% [ cos(psi)*sin(theta) + cos(theta)*sin(phi)*sin(psi), 
%     sin(psi)*sin(theta) - cos(psi)*cos(theta)*sin(phi),
%     cos(phi)*cos(theta)]

R = [ cos(psi)*cos(theta) - sin(phi)*sin(psi)*sin(theta),... 
    cos(theta)*sin(psi) + cos(psi)*sin(phi)*sin(theta), -cos(phi)*sin(theta);...
    -cos(phi)*sin(psi),...
    cos(phi)*cos(psi),             sin(phi);...
    cos(psi)*sin(theta) + cos(theta)*sin(phi)*sin(psi),...
    sin(psi)*sin(theta) - cos(psi)*cos(theta)*sin(phi),...
    cos(phi)*cos(theta)];
    
    R = R';

== matlab function multi_model_attitude_controller1_1/control_system/Subsystem/MATLAB Function5 ==
  data: RdR_RRd input; err_R output
function err_R = vee(RdR_RRd)
%     if(nargin == 1)
%         force = false ;
%     end
%     if(~force)
%         if(double(sum(abs(diag(A)))) > 1e-2)
%             disp('Error in vee_map() - Nonzero diagonal') ;
% %             keyboard ;
%         end
%     end
    %A = [0 -t(3) t(2) ; t(3) 0 -t(1) ; -t(2) t(1) 0] ;
    err_R = [RdR_RRd(3,2) ;
         RdR_RRd(1,3) ;
         RdR_RRd(2,1)] ;
end

== matlab function multi_model_attitude_controller1_1/control_system/Subsystem3/Subsystem/MATLAB Function1 ==
  data: phi input; R output; theta input; psi input
function R = RPYtoRot_ZXY(phi,theta,psi)
%written by Daniel Mellinger

% BRW = [ cos(psi)*cos(theta) - sin(phi)*sin(psi)*sin(theta), 
%     cos(theta)*sin(psi) + cos(psi)*sin(phi)*sin(theta), -cos(phi)*sin(theta)]
% 
% [                                 -cos(phi)*sin(psi),
%     cos(phi)*cos(psi),             sin(phi)]
% 
% [ cos(psi)*sin(theta) + cos(theta)*sin(phi)*sin(psi), 
%     sin(psi)*sin(theta) - cos(psi)*cos(theta)*sin(phi),
%     cos(phi)*cos(theta)]

R = [ cos(psi)*cos(theta) - sin(phi)*sin(psi)*sin(theta),... 
    cos(theta)*sin(psi) + cos(psi)*sin(phi)*sin(theta), -cos(phi)*sin(theta);...
    -cos(phi)*sin(psi),...
    cos(phi)*cos(psi),             sin(phi);...
    cos(psi)*sin(theta) + cos(theta)*sin(phi)*sin(psi),...
    sin(psi)*sin(theta) - cos(psi)*cos(theta)*sin(phi),...
    cos(phi)*cos(theta)];
    
    R = R';

== matlab function multi_model_attitude_controller1_1/control_system/Subsystem/MATLAB Function7 ==
  data: a input; RR output; b input
function RR = a_b(a,b)
RR = a'*b ;

== matlab function multi_model_attitude_controller1_1/control_system/Subsystem/MATLAB Function8 ==
  data: a input; RR output; b input
function RR = a_b(a,b)
RR = a'*b ;

== matlab function multi_model_attitude_controller1_1/control_system/Subsystem3/Subsystem/MATLAB Function3 ==
  data: R input; phi output; theta output; psi output
function [phi,theta,psi] = RotToRPY_ZXY(R)
%written by Daniel Mellinger

% 
% R = [ cos(psi)*cos(theta) - sin(phi)*sin(psi)*sin(theta), 
%     cos(theta)*sin(psi) + cos(psi)*sin(phi)*sin(theta), -cos(phi)*sin(theta)]
% 
% [                                 -cos(phi)*sin(psi),
%     cos(phi)*cos(psi),             sin(phi)]
% 
% [ cos(psi)*sin(theta) + cos(theta)*sin(phi)*sin(psi), 
%     sin(psi)*sin(theta) - cos(psi)*cos(theta)*sin(phi),  cos(phi)*cos(theta)]
R = R';
phi = asin(R(2,3));
psi = atan2(-R(2,1)/cos(phi),R(2,2)/cos(phi));
theta = atan2(-R(1,3)/cos(phi),R(3,3)/cos(phi));

== matlab function multi_model_attitude_controller1_1/control_system/Subsystem3/MATLAB Function4 ==
  data: R input; phi output; theta output; psi output
function [phi,theta,psi] = RotToRPY_ZXY(R)
%written by Daniel Mellinger

% 
% R = [ cos(psi)*cos(theta) - sin(phi)*sin(psi)*sin(theta), 
%     cos(theta)*sin(psi) + cos(psi)*sin(phi)*sin(theta), -cos(phi)*sin(theta)]
% 
% [                                 -cos(phi)*sin(psi),
%     cos(phi)*cos(psi),             sin(phi)]
% 
% [ cos(psi)*sin(theta) + cos(theta)*sin(phi)*sin(psi), 
%     sin(psi)*sin(theta) - cos(psi)*cos(theta)*sin(phi),  cos(phi)*cos(theta)]
R = R';
phi = asin(R(2,3));
psi = atan2(-R(2,1)/cos(phi),R(2,2)/cos(phi));
theta = atan2(-R(1,3)/cos(phi),R(3,3)/cos(phi));

== matlab function multi_model_attitude_controller1_1/control_system/Subsystem3/MATLAB Function1 ==
  data: phi input; R output; theta input; psi input
function R = RPYtoRot_ZXY(phi,theta,psi)
%written by Daniel Mellinger

% BRW = [ cos(psi)*cos(theta) - sin(phi)*sin(psi)*sin(theta), 
%     cos(theta)*sin(psi) + cos(psi)*sin(phi)*sin(theta), -cos(phi)*sin(theta)]
% 
% [                                 -cos(phi)*sin(psi),
%     cos(phi)*cos(psi),             sin(phi)]
% 
% [ cos(psi)*sin(theta) + cos(theta)*sin(phi)*sin(psi), 
%     sin(psi)*sin(theta) - cos(psi)*cos(theta)*sin(phi),
%     cos(phi)*cos(theta)]

R = [ cos(psi)*cos(theta) - sin(phi)*sin(psi)*sin(theta),... 
    cos(theta)*sin(psi) + cos(psi)*sin(phi)*sin(theta), -cos(phi)*sin(theta);...
    -cos(phi)*sin(psi),...
    cos(phi)*cos(psi),             sin(phi);...
    cos(psi)*sin(theta) + cos(theta)*sin(phi)*sin(psi),...
    sin(psi)*sin(theta) - cos(psi)*cos(theta)*sin(phi),...
    cos(phi)*cos(theta)];
    
    R = R';

== matlab function multi_model_attitude_controller1_1/dynamic_model1/LiPo Battery ==
  data: load input; voltage output; cell_voltage output
function [voltage, cell_voltage]= LiPo(load)

%================================Constants=================================

delta_t = 0.004;
max_current = 5.500;                % maximum current per motor             (A)
aux_current = 0.100;                % current of auxillary components       (A)        
capacity = 1.000;                   % LiPo current capacity                 (Ah)                                 
cells = 2;                          % LiPo cell count

%==========================================================================

persistent discharge;

if isempty(discharge)
    discharge = 0;
end

current = sum(max_current .* load.^2) + aux_current;
discharge = current * (delta_t / 3600) + discharge;

discharge_capacity = discharge / capacity;

if (0 < discharge_capacity) && (discharge_capacity <=0.20)
    cell_voltage = -14.029*discharge_capacity^3 + 16.975*discharge_capacity^2 - 5.3339*discharge_capacity + 4.2;
elseif (0.20 < discharge_capacity) && (discharge_capacity < 0.70)
    cell_voltage = -0.2*discharge_capacity + 3.74;
else
    cell_voltage = -48*discharge_capacity^3 + 89.6*discharge_capacity^2 - 55.08*discharge_capacity + 14.716;
end

if cell_voltage < (5 / cells)
    cell_voltage = 0;
end
cell_voltage = 4.2;
supply_voltage = cells * cell_voltage;
voltage = supply_voltage .* load;

%==========================================================================

== matlab function multi_model_attitude_controller1_1/dynamic_model1/MATLAB Function ==
  data: roll input; pitch input; altitude input; sonar_alt output
function sonar_alt = ultrasonic(roll, pitch, altitude)
if altitude > 0
    sonar_alt = sqrt(altitude^2 + (sqrt((altitude*tan(roll))^2 + (altitude*tan(pitch))^2))^2);
else
    sonar_alt = 0;
end

== matlab function multi_model_attitude_controller1_1/dynamic_model1/multicopter ==
  data: omega input; DCM input; velocity input; density input; rotors input; forces output; moments output
function [forces, moments] = multicopter(omega, DCM, velocity, density, rotors)

%================================Constants=================================

coefficient_drag = 15;              % coefficient of drag
rotor_inertia = 0.0000025;          % rotor inertia                         (kg m^2)
prop_diameter = 0.1397;             % diameter of the propellor             (meters)                                 
% aircraft_mass = 0.26;               % aircraft mass                         (kg) 
aircraft_mass = 0.26; 
aircraft_diameter = 0.25;           % motor to motor distance               (meters)                                      

%==============================Actuator Mixer==============================

% [x(roll), y(pitch), z(yaw)]


MIX = [  1   1  -1   ;      % QUAD [X]
        -1   1   1   ;
        -1  -1  -1   ;
         1  -1   1   ;
         0   0   0   ;
         0   0   0   ;
         0   0   0   ;
         0   0   0   ];

% MIX = [  0   1  -1   ;      % QUAD [+]
%         -1   0   1   ;
%          0  -1  -1   ;
%          1   0   1   ;
%          0   0   0   ;
%          0   0   0   ;
%          0   0   0   ;
%          0   0   0   ];

% MIX = [  1   1  -1   ;      % HEX [X]
%         -1   1   1   ;
%         -1   0  -1   ;
%         -1  -1   1   ;
%          1  -1  -1   ;
%          1   0   1   ;
%          0   0   0   ;
%          0   0   0   ];

%==================================Forces================================== 

a = [   aircraft_diameter^2 / 10                        ;...                % body cross sectional area (X)
        aircraft_diameter^2 / 10                        ;...                % body cross sectional area (Y)
        sum(abs(MIX(:, 3))) * pi/4 * prop_diameter^2    ];                  % body cross sectional area (Z)
    
gravity = aircraft_mass .* (DCM * [0; 0; 9.81]);                            % gravitational force
% drag = -velocity .* coefficient_drag .* density .* a;                       % drag force
drag = [0;0;0];
%--------------------------------Thrust Model------------------------------
thrust = abs(MIX(:, 3)) .* (1*1E-3) .* rotors;                              % rotor thrust <==     
%--------------------------------------------------------------------------

forces = gravity + drag;
forces(3) = forces(3) - sum(thrust);

%==================================Moments=================================

mx = thrust .* MIX(:,1) .* (aircraft_diameter / 2)*sind(45);                % x moment
my = thrust .* MIX(:,2) .* (aircraft_diameter / 2)*sind(45);                % y moment

momentum_x = sum(abs(MIX(:, 3)) .* rotor_inertia .* rotors) * omega(1);     % x rotor momentum
momentum_y = sum(abs(MIX(:, 3)) .* rotor_inertia .* rotors) * omega(2);     % y rotor momentum
momentum_z = sum(MIX(:, 3) .* rotor_inertia .* rotors) * omega(3);          % z rotor momentum

%--------------------------------Torque Model------------------------------
mz = MIX(:,3) .* (1.7E-5) .* rotors;                                        % rotor torque <==
%--------------------------------------------------------------------------

% moments = [sum(mx); sum(my); sum(mz)] - [momentum_x; momentum_y;
% momentum_z];%%momented by yike
moments = [sum(mx); sum(my); sum(mz)];%%added by yike

%==========================================================================

== matlab function multi_model_attitude_controller1_1/control_system1/Subsystem/MATLAB Function5 ==
  data: RdR_RRd input; err_R output
function err_R = vee(RdR_RRd)
%     if(nargin == 1)
%         force = false ;
%     end
%     if(~force)
%         if(double(sum(abs(diag(A)))) > 1e-2)
%             disp('Error in vee_map() - Nonzero diagonal') ;
% %             keyboard ;
%         end
%     end
    %A = [0 -t(3) t(2) ; t(3) 0 -t(1) ; -t(2) t(1) 0] ;
    err_R = [RdR_RRd(3,2) ;
         RdR_RRd(1,3) ;
         RdR_RRd(2,1)] ;
end

== matlab function multi_model_attitude_controller1_1/control_system1/Subsystem/MATLAB Function7 ==
  data: a input; RR output; b input
function RR = a_b(a,b)
RR = a'*b ;

== matlab function multi_model_attitude_controller1_1/control_system1/Subsystem/MATLAB Function8 ==
  data: a input; RR output; b input
function RR = a_b(a,b)
RR = a'*b ;

== matlab function multi_model_attitude_controller1_1/control_system1/Subsystem1/MATLAB Function2 ==
  data: A input; M_roll output; angular_c input; angular_velocity_c input; M_pitch output; M_yaw output; u1 output; rolld output; pitchd output; yawd output; angular_d input; disturbance input
function [M_roll, M_pitch,M_yaw,u1,rolld,pitchd,yawd] = attitude(A,angular_c,angular_velocity_c,angular_d,disturbance)

 J = diag([0.00080, 0.00065, 0.0014]);
 e1 = [1;0;0];e2 = [0;1;0];e3 = [0;0;1];
%%当前状态量
roll=angular_c(1);pitch=angular_c(2);yaw=angular_c(3);

R= RPYtoRot_ZXY(roll,pitch,yaw);
Omega=angular_velocity_c;

 b3c = A/norm(A);
 b3 = R(:,3);
 f = vec_dot(A,b3);
 u1=f;
    
%%%%%  姿态控制
 b1d = e1;
 b1c = -vec_cross(b3c,vec_cross(b3c,b1d));
 b1c = b1c/norm(vec_cross(b3c,b1d));
 Rc = [b1c vec_cross(b3c,b1c) b3c];
 
roll_d=pi/4;
pitch_d=-pi/4;
yaw_d=0;

roll_d=angular_d(1);
pitch_d=angular_d(2);
yaw_d=angular_d(3);

Rc= RPYtoRot_ZXY(roll_d,pitch_d,yaw_d);
Rd = Rc;
[rolld,pitchd,yawd]=RotToRPY_ZXY(Rd);
 if(norm(Rd'*Rd-eye(3)) > 1e-2)
        disp('Error in R') ;
 end

%  kR = 0.4 ; kOm = 0.4 ;
%   kR = 3	 ; kOm =2 ;
%   kR = 0.09	 ; kOm =1 ;
kR = 4	 ; kOm =1 ;
% epsilon = 0.1 ; %.5 ; %0.01 ;
Omegad = zeros(3,1);
dOmegad = zeros(3,1);
err_R = 1/2 * vee_map(Rd'*R - R'*Rd) ;
err_Om = Omega - R'*Rd*Omegad ;
 
% M = -kR.*err_R - kOm.*err_Om+ vec_cross(Omega, J*Omega)- J*(hat_map(Omega)*R'*Rd*Omegad - R'*Rd*dOmegad) ;
M = -kR.*err_R - kOm.*err_Om+ vec_cross(Omega, J*Omega)- J*(hat_map(Omega)*R'*Rd*Omegad - R'*Rd*dOmegad)-(disturbance) ;
M_roll=M(1);M_pitch=M(2);M_yaw=M(3);
% M_phi=0 ;M_theta=0;M_psi=0;
% M_pitch=0;
% % M_roll=0 ;
% M_yaw=0;
% u1=0.5;

== matlab function multi_model_attitude_controller1_1/control_system1/Subsystem3/MATLAB Function1 ==
  data: phi input; R output; theta input; psi input
function R = RPYtoRot_ZXY(phi,theta,psi)
%written by Daniel Mellinger

% BRW = [ cos(psi)*cos(theta) - sin(phi)*sin(psi)*sin(theta), 
%     cos(theta)*sin(psi) + cos(psi)*sin(phi)*sin(theta), -cos(phi)*sin(theta)]
% 
% [                                 -cos(phi)*sin(psi),
%     cos(phi)*cos(psi),             sin(phi)]
% 
% [ cos(psi)*sin(theta) + cos(theta)*sin(phi)*sin(psi), 
%     sin(psi)*sin(theta) - cos(psi)*cos(theta)*sin(phi),
%     cos(phi)*cos(theta)]

R = [ cos(psi)*cos(theta) - sin(phi)*sin(psi)*sin(theta),... 
    cos(theta)*sin(psi) + cos(psi)*sin(phi)*sin(theta), -cos(phi)*sin(theta);...
    -cos(phi)*sin(psi),...
    cos(phi)*cos(psi),             sin(phi);...
    cos(psi)*sin(theta) + cos(theta)*sin(phi)*sin(psi),...
    sin(psi)*sin(theta) - cos(psi)*cos(theta)*sin(phi),...
    cos(phi)*cos(theta)];
    
    R = R';

== matlab function multi_model_attitude_controller1_1/control_system1/Subsystem3/MATLAB Function2 ==
  data: A input; M_roll output; R input; angular_velocity_c input; M_pitch output; M_yaw output; u1 output; rolld output; pitchd output; yawd output; Rd output; kR output; kOm output; Rd input; err_R output; err_Om output; rated input; ratedd input; psi_attract output
function [M_roll, M_pitch,M_yaw,u1,rolld,pitchd,yawd,Rd,kR,kOm,err_R,err_Om,psi_attract] = attitude(A,R,angular_velocity_c,Rd,rated,ratedd)

 J = diag([0.00080, 0.00065, 0.0014]);
 J_ni=inv(J);
 e1 = [1;0;0];e2 = [0;1;0];e3 = [0;0;1];

Omega=angular_velocity_c;

Omegad = rated;
dOmegad = ratedd;

 b3c = A/norm(A);
 b3 = R(:,3);
 f = vec_dot(A,b3);
 u1=f;
    
%%%%%  姿态控制
 b1d = e1;
 b1c = -vec_cross(b3c,vec_cross(b3c,b1d));
 b1c = b1c/norm(vec_cross(b3c,b1d));
 Rc = [b1c vec_cross(b3c,b1c) b3c];
 

[rolld,pitchd,yawd]=RotToRPY_ZXY(Rd);
 if(norm(Rd'*Rd-eye(3)) > 1e-2)
        disp('Error in R') ;
 end

%  kR = 0.4 ; kOm = 0.4 ;
%   kR = 3	 ; kOm =2 ;
%   kR = 0.09	 ; kOm =1 ;
kR = 0.5	 ; kOm =0.005;
% epsilon = 0.1 ; %.5 ; %0.01 ;

psi_attract = 1/2*trace(eye(3,3)-Rd'*R);
err_R = 1/2 * vee_map(Rd'*R - R'*Rd) ;
err_Om = Omega - R'*Rd*Omegad ;
 

% % kR=0.1.*kR+err_R'*err_Om;
% % if kR>1
% %     kR=1;
% % end
% % if kR<-1
% %     kR=-1;
% % end
% % 
% % kOm=0.1.*kOm+0.01.*err_R'*err_Om;
% % if kOm>0.5
% %     kOm=0.5;
% % end
% % if kOm<-0.5
% %     kOm=0-0.5;
% % end

c2=0.02;
eA=err_Om+c2.*J_ni*err_R;
deltaR=0.3;
sigamaR=0.01;
k=0.1;

miu=-(deltaR.^2+k.*sigamaR).*eA./(deltaR*norm(eA)+sigamaR);
% miu=[0;0;0];


M = -kR.*err_R - kOm.*err_Om+ vec_cross(Omega, J*Omega)- J*(hat_map(Omega)*R'*Rd*Omegad - R'*Rd*dOmegad)+miu ;
% % M = -kR.*err_R - kOm.*err_Om+miu ;
M_roll=M(1);M_pitch=M(2);M_yaw=M(3);

== matlab function multi_model_attitude_controller1_1/control_system1/Subsystem3/MATLAB Function4 ==
  data: R input; phi output; theta output; psi output
function [phi,theta,psi] = RotToRPY_ZXY(R)
%written by Daniel Mellinger

% 
% R = [ cos(psi)*cos(theta) - sin(phi)*sin(psi)*sin(theta), 
%     cos(theta)*sin(psi) + cos(psi)*sin(phi)*sin(theta), -cos(phi)*sin(theta)]
% 
% [                                 -cos(phi)*sin(psi),
%     cos(phi)*cos(psi),             sin(phi)]
% 
% [ cos(psi)*sin(theta) + cos(theta)*sin(phi)*sin(psi), 
%     sin(psi)*sin(theta) - cos(psi)*cos(theta)*sin(phi),  cos(phi)*cos(theta)]
R = R';
phi = asin(R(2,3));
psi = atan2(-R(2,1)/cos(phi),R(2,2)/cos(phi));
theta = atan2(-R(1,3)/cos(phi),R(3,3)/cos(phi));

== matlab function multi_model_attitude_controller1_1/control_system1/Subsystem3/Subsystem/MATLAB Function1 ==
  data: phi input; R output; theta input; psi input
function R = RPYtoRot_ZXY(phi,theta,psi)
%written by Daniel Mellinger

% BRW = [ cos(psi)*cos(theta) - sin(phi)*sin(psi)*sin(theta), 
%     cos(theta)*sin(psi) + cos(psi)*sin(phi)*sin(theta), -cos(phi)*sin(theta)]
% 
% [                                 -cos(phi)*sin(psi),
%     cos(phi)*cos(psi),             sin(phi)]
% 
% [ cos(psi)*sin(theta) + cos(theta)*sin(phi)*sin(psi), 
%     sin(psi)*sin(theta) - cos(psi)*cos(theta)*sin(phi),
%     cos(phi)*cos(theta)]

R = [ cos(psi)*cos(theta) - sin(phi)*sin(psi)*sin(theta),... 
    cos(theta)*sin(psi) + cos(psi)*sin(phi)*sin(theta), -cos(phi)*sin(theta);...
    -cos(phi)*sin(psi),...
    cos(phi)*cos(psi),             sin(phi);...
    cos(psi)*sin(theta) + cos(theta)*sin(phi)*sin(psi),...
    sin(psi)*sin(theta) - cos(psi)*cos(theta)*sin(phi),...
    cos(phi)*cos(theta)];
    
    R = R';

== matlab function multi_model_attitude_controller1_1/control_system1/Subsystem3/Subsystem/MATLAB Function3 ==
  data: R input; phi output; theta output; psi output
function [phi,theta,psi] = RotToRPY_ZXY(R)
%written by Daniel Mellinger

% 
% R = [ cos(psi)*cos(theta) - sin(phi)*sin(psi)*sin(theta), 
%     cos(theta)*sin(psi) + cos(psi)*sin(phi)*sin(theta), -cos(phi)*sin(theta)]
% 
% [                                 -cos(phi)*sin(psi),
%     cos(phi)*cos(psi),             sin(phi)]
% 
% [ cos(psi)*sin(theta) + cos(theta)*sin(phi)*sin(psi), 
%     sin(psi)*sin(theta) - cos(psi)*cos(theta)*sin(phi),  cos(phi)*cos(theta)]
R = R';
phi = asin(R(2,3));
psi = atan2(-R(2,1)/cos(phi),R(2,2)/cos(phi));
theta = atan2(-R(1,3)/cos(phi),R(3,3)/cos(phi));

== matlab function multi_model_attitude_controller1_1/control_system1/Subsystem3/Subsystem/MATLAB Function5 ==
  data: A input; t output; force input
function t = vee_map(A, force)
    if(nargin == 1)
        force = false ;
    end
    if(~force)
        if(double(sum(abs(diag(A)))) > 1e-2)
            disp('Error in vee_map() - Nonzero diagonal') ;
%             keyboard ;
        end
    end
    %A = [0 -t(3) t(2) ; t(3) 0 -t(1) ; -t(2) t(1) 0] ;
    t = [A(3,2) ;
         A(1,3) ;
         A(2,1)] ;
end
